simulink library "afa"  (Simulink 8.1)
settings: Solver=ode45  StartTime=0.0  StopTime=10.0  RelTol=1e-3
undefined symbols (not defined in the file or in its folder): ENUM_FCWSTATE_DBS, FALSE, KFCW_DefaultDBSDecel_mps2, KFCW_HapticOnDecelVal_mps2, KFCW_HoldModeLimitSpeed_kph, KFCW_MaxDBSDeceleration_mps2, KFCW_MinDBSDeceleration_mps2, KFCW_WarnLightsDecel_mps2, KFCW_WarnLightSpeedThresh_kph, ZERO_FLOAT
libraries: hcu_lib x2
settings Model: Creator=xsellart  LastModifiedBy=tescamilla

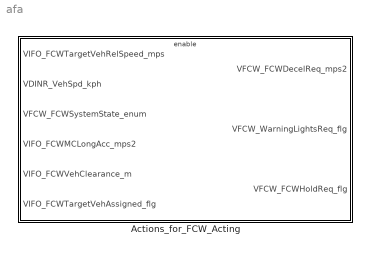
== system afa ==
  Actions_for_FCW_Acting : Subsystem  TreatAsAtomicUnit=on

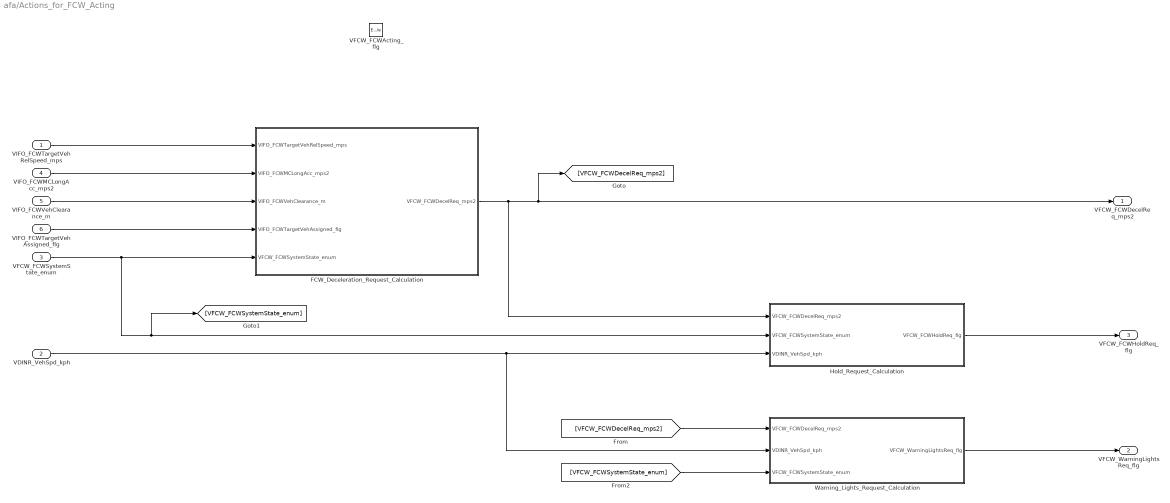
== system afa/Actions_for_FCW_Acting ==
  VIFO_FCWTargetVehRelSpeed_mps : Inport
  VDINR_VehSpd_kph : Inport  Port=2
  VFCW_FCWSystemState_enum : Inport  Port=3
  VIFO_FCWMCLongAcc_mps2 : Inport  Port=4
  VIFO_FCWVehClearance_m : Inport  Port=5
  VIFO_FCWTargetVehAssigned_flg : Inport  Port=6
  VFCW_FCWActing_flg : EnablePort  StatesWhenEnabling=reset
      settings: AttributesFormatString=State=%<StatesWhenEnabling>
  FCW_Deceleration_Request_Calculation : Subsystem
  Hold_Request_Calculation : Subsystem
  Warning_Lights_Request_Calculation : Subsystem
  VFCW_FCWDecelReq_mps2 : Outport  OutputWhenDisabled=reset  InitialOutput=ZERO_FLOAT
  VFCW_WarningLightsReq_flg : Outport  Port=2  OutputWhenDisabled=reset  InitialOutput=FALSE
  VFCW_FCWHoldReq_flg : Outport  Port=3  OutputWhenDisabled=reset  InitialOutput=FALSE
  wires:
  Warning_Lights_Request_Calculation/1(VFCW_WarningLightsReq_flg) -> VFCW_WarningLightsReq_flg/1
  VDINR_VehSpd_kph/1 -> Warning_Lights_Request_Calculation/2(VDINR_VehSpd_kph), Hold_Request_Calculation/3(VDINR_VehSpd_kph)
  VIFO_FCWTargetVehRelSpeed_mps/1 -> FCW_Deceleration_Request_Calculation/1(VIFO_FCWTargetVehRelSpeed_mps)
  Hold_Request_Calculation/1(VFCW_FCWHoldReq_flg) -> VFCW_FCWHoldReq_flg/1
  FCW_Deceleration_Request_Calculation/1(VFCW_FCWDecelReq_mps2) -> VFCW_FCWDecelReq_mps2/1, [VFCW_FCWDecelReq_mps2], Hold_Request_Calculation/1(VFCW_FCWDecelReq_mps2)
  VFCW_FCWSystemState_enum/1 -> [VFCW_FCWSystemState_enum], Hold_Request_Calculation/2(VFCW_FCWSystemState_enum), FCW_Deceleration_Request_Calculation/5(VFCW_FCWSystemState_enum)
  [VFCW_FCWDecelReq_mps2] -> Warning_Lights_Request_Calculation/1(VFCW_FCWDecelReq_mps2)
  [VFCW_FCWSystemState_enum] -> Warning_Lights_Request_Calculation/3(VFCW_FCWSystemState_enum)
  VIFO_FCWMCLongAcc_mps2/1 -> FCW_Deceleration_Request_Calculation/2(VIFO_FCWMCLongAcc_mps2)
  VIFO_FCWVehClearance_m/1 -> FCW_Deceleration_Request_Calculation/3(VIFO_FCWVehClearance_m)
  VIFO_FCWTargetVehAssigned_flg/1 -> FCW_Deceleration_Request_Calculation/4(VIFO_FCWTargetVehAssigned_flg)

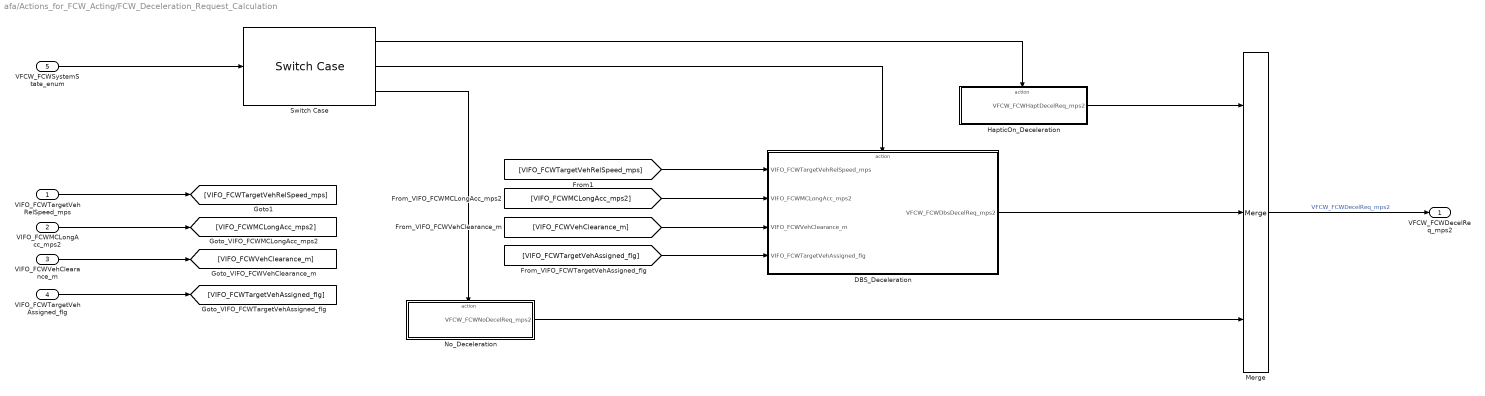
== system afa/Actions_for_FCW_Acting/FCW_Deceleration_Request_Calculation ==
  VIFO_FCWTargetVehRelSpeed_mps : Inport
  VIFO_FCWMCLongAcc_mps2 : Inport  Port=2
  VIFO_FCWVehClearance_m : Inport  Port=3
  VIFO_FCWTargetVehAssigned_flg : Inport  Port=4
  VFCW_FCWSystemState_enum : Inport  Port=5
  DBS_Deceleration : Subsystem  TreatAsAtomicUnit=on
  HapticOn_Deceleration : Subsystem  TreatAsAtomicUnit=on
  Merge : Merge  Inputs=3
  No_Deceleration : Subsystem  TreatAsAtomicUnit=on
  Switch Case : SwitchCase  CaseConditions={5, 7}
  VFCW_FCWDecelReq_mps2 : Outport  OutDataTypeStr=single
  wires:
  VFCW_FCWSystemState_enum/1 -> Switch Case/1
  Switch Case/1 -> HapticOn_Deceleration/Action
  Switch Case/2 -> DBS_Deceleration/Action
  VIFO_FCWTargetVehRelSpeed_mps/1 -> [VIFO_FCWTargetVehRelSpeed_mps]
  [VIFO_FCWTargetVehRelSpeed_mps] -> DBS_Deceleration/1(VIFO_FCWTargetVehRelSpeed_mps)
  Switch Case/3 -> No_Deceleration/Action
  HapticOn_Deceleration/1(VFCW_FCWHaptDecelReq_mps2) -> Merge/1
  DBS_Deceleration/1(VFCW_FCWDbsDecelReq_mps2) -> Merge/2
  No_Deceleration/1(VFCW_FCWNoDecelReq_mps2) -> Merge/3
  Merge/1 -> VFCW_FCWDecelReq_mps2/1  "VFCW_FCWDecelReq_mps2"
  [VIFO_FCWMCLongAcc_mps2] -> DBS_Deceleration/2(VIFO_FCWMCLongAcc_mps2)
  VIFO_FCWMCLongAcc_mps2/1 -> [VIFO_FCWMCLongAcc_mps2]
  VIFO_FCWVehClearance_m/1 -> [VIFO_FCWVehClearance_m]
  [VIFO_FCWVehClearance_m] -> DBS_Deceleration/3(VIFO_FCWVehClearance_m)
  [VIFO_FCWTargetVehAssigned_flg] -> DBS_Deceleration/4(VIFO_FCWTargetVehAssigned_flg)
  VIFO_FCWTargetVehAssigned_flg/1 -> [VIFO_FCWTargetVehAssigned_flg]

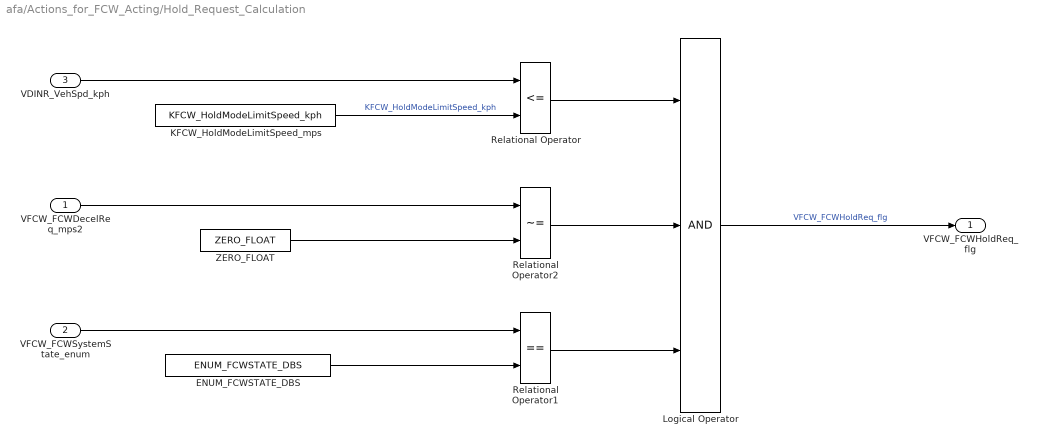
== system afa/Actions_for_FCW_Acting/Hold_Request_Calculation ==
  VFCW_FCWDecelReq_mps2 : Inport
  VFCW_FCWSystemState_enum : Inport  Port=2
  VDINR_VehSpd_kph : Inport  Port=3
  ENUM_FCWSTATE_DBS : Constant  Value=ENUM_FCWSTATE_DBS  OutDataTypeStr=uint8
  KFCW_HoldModeLimitSpeed_mps : Constant  Value=KFCW_HoldModeLimitSpeed_kph  OutDataTypeStr=single
  Logical Operator : Logic  Inputs=3  AllPortsSameDT=off  OutDataTypeStr=boolean
  Relational Operator : RelationalOperator  Operator=<=  OutDataTypeStr=boolean
  Relational Operator1 : RelationalOperator  Operator===  OutDataTypeStr=boolean
  Relational Operator2 : RelationalOperator  Operator=~=  OutDataTypeStr=boolean
  ZERO_FLOAT : Constant  Value=ZERO_FLOAT  OutDataTypeStr=single
  VFCW_FCWHoldReq_flg : Outport
  wires:
  KFCW_HoldModeLimitSpeed_mps/1 -> Relational Operator/2  "KFCW_HoldModeLimitSpeed_kph"
  VDINR_VehSpd_kph/1 -> Relational Operator/1
  ENUM_FCWSTATE_DBS/1 -> Relational Operator1/2
  VFCW_FCWSystemState_enum/1 -> Relational Operator1/1
  Relational Operator2/1 -> Logical Operator/2
  Relational Operator1/1 -> Logical Operator/3
  Logical Operator/1 -> VFCW_FCWHoldReq_flg/1  "VFCW_FCWHoldReq_flg"
  ZERO_FLOAT/1 -> Relational Operator2/2
  VFCW_FCWDecelReq_mps2/1 -> Relational Operator2/1
  Relational Operator/1 -> Logical Operator/1

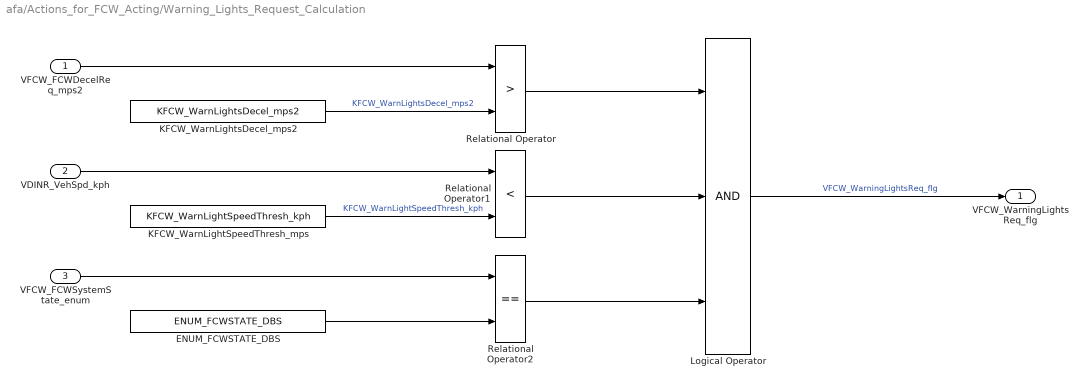
== system afa/Actions_for_FCW_Acting/Warning_Lights_Request_Calculation ==
  VFCW_FCWDecelReq_mps2 : Inport
  VDINR_VehSpd_kph : Inport  Port=2
  VFCW_FCWSystemState_enum : Inport  Port=3
  ENUM_FCWSTATE_DBS : Constant  Value=ENUM_FCWSTATE_DBS  OutDataTypeStr=uint8
  KFCW_WarnLightSpeedThresh_mps : Constant  Value=KFCW_WarnLightSpeedThresh_kph
  KFCW_WarnLightsDecel_mps2 : Constant  Value=KFCW_WarnLightsDecel_mps2
  Logical Operator : Logic  Inputs=3  AllPortsSameDT=off  OutDataTypeStr=boolean
  Relational Operator : RelationalOperator  Operator=>  OutDataTypeStr=boolean
  Relational Operator1 : RelationalOperator  Operator=<  OutDataTypeStr=boolean
  Relational Operator2 : RelationalOperator  Operator===  OutDataTypeStr=boolean
  VFCW_WarningLightsReq_flg : Outport  OutputWhenDisabled=reset  InitialOutput=FALSE
  wires:
  KFCW_WarnLightsDecel_mps2/1 -> Relational Operator/2  "KFCW_WarnLightsDecel_mps2"
  VFCW_FCWDecelReq_mps2/1 -> Relational Operator/1
  KFCW_WarnLightSpeedThresh_mps/1 -> Relational Operator1/2  "KFCW_WarnLightSpeedThresh_kph"
  VDINR_VehSpd_kph/1 -> Relational Operator1/1
  Relational Operator/1 -> Logical Operator/1
  Relational Operator1/1 -> Logical Operator/2
  Logical Operator/1 -> VFCW_WarningLightsReq_flg/1  "VFCW_WarningLightsReq_flg"
  VFCW_FCWSystemState_enum/1 -> Relational Operator2/1
  ENUM_FCWSTATE_DBS/1 -> Relational Operator2/2
  Relational Operator2/1 -> Logical Operator/3

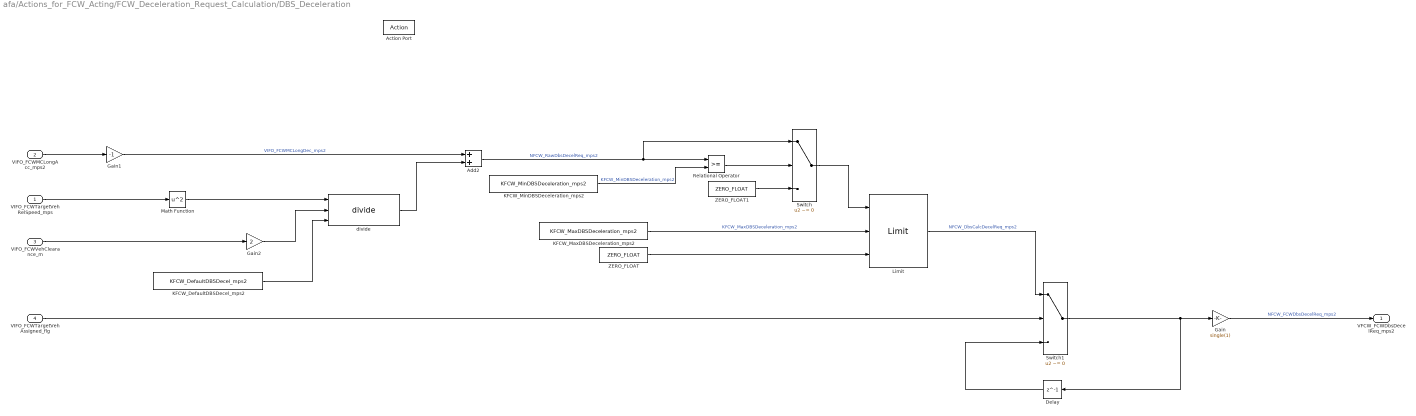
== system afa/Actions_for_FCW_Acting/FCW_Deceleration_Request_Calculation/DBS_Deceleration ==
  VIFO_FCWTargetVehRelSpeed_mps : Inport
  VIFO_FCWMCLongAcc_mps2 : Inport  Port=2
  VIFO_FCWVehClearance_m : Inport  Port=3
  VIFO_FCWTargetVehAssigned_flg : Inport  Port=4
  Action Port : ActionPort  ActionType=case
  Add2 : Sum
  Delay : Delay  DelayLength=1  InitialCondition=0
  Gain : Gain  Gain=single(1)
  Gain1 : Gain  Gain=-1
  Gain2 : Gain  Gain=2
  KFCW_DefaultDBSDecel_mps2 : Constant  Value=KFCW_DefaultDBSDecel_mps2
  KFCW_MaxDBSDeceleration_mps2 : Constant  Value=KFCW_MaxDBSDeceleration_mps2
  KFCW_MinDBSDeceleration_mps2 : Constant  Value=KFCW_MinDBSDeceleration_mps2
  Limit : hcu_lib/Limit  SystemSampleTime=-1
  Math Function : Math  Operator=square  SaturateOnIntegerOverflow=on
  Relational Operator : RelationalOperator  OutDataTypeStr=boolean
  Switch : Switch  Criteria=u2 ~= 0
  Switch1 : Switch  Criteria=u2 ~= 0
  ZERO_FLOAT : Constant  Value=ZERO_FLOAT
  ZERO_FLOAT1 : Constant  Value=ZERO_FLOAT
  divide : hcu_lib/divide
  VFCW_FCWDbsDecelReq_mps2 : Outport
  wires:
  ZERO_FLOAT/1 -> Limit/3
  VIFO_FCWTargetVehRelSpeed_mps/1 -> Math Function/1
  KFCW_MaxDBSDeceleration_mps2/1 -> Limit/2  "KFCW_MaxDBSDeceleration_mps2"
  Limit/1 -> Switch1/1  "NFCW_DbsCalcDecelReq_mps2"
  VIFO_FCWMCLongAcc_mps2/1 -> Gain1/1
  Math Function/1 -> divide/1
  VIFO_FCWVehClearance_m/1 -> Gain2/1
  Gain2/1 -> divide/2
  KFCW_DefaultDBSDecel_mps2/1 -> divide/3
  Gain1/1 -> Add2/1  "VIFO_FCWMCLongDec_mps2"
  divide/1 -> Add2/2
  Add2/1 -> Switch/1, Relational Operator/1  "NFCW_RawDbsDecelReq_mps2"
  KFCW_MinDBSDeceleration_mps2/1 -> Relational Operator/2  "KFCW_MinDBSDeceleration_mps2"
  Relational Operator/1 -> Switch/2
  ZERO_FLOAT1/1 -> Switch/3
  Switch/1 -> Limit/1
  VIFO_FCWTargetVehAssigned_flg/1 -> Switch1/2
  Switch1/1 -> Delay/1, Gain/1
  Delay/1 -> Switch1/3
  Gain/1 -> VFCW_FCWDbsDecelReq_mps2/1  "NFCW_FCWDbsDecelReq_mps2"

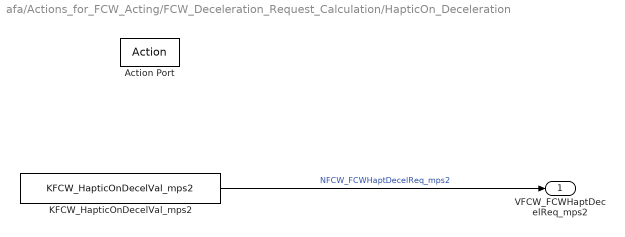
== system afa/Actions_for_FCW_Acting/FCW_Deceleration_Request_Calculation/HapticOn_Deceleration ==
  Action Port : ActionPort  ActionType=case
  KFCW_HapticOnDecelVal_mps2 : Constant  Value=KFCW_HapticOnDecelVal_mps2  OutDataTypeStr=single
  VFCW_FCWHaptDecelReq_mps2 : Outport
  wires:
  KFCW_HapticOnDecelVal_mps2/1 -> VFCW_FCWHaptDecelReq_mps2/1  "NFCW_FCWHaptDecelReq_mps2"

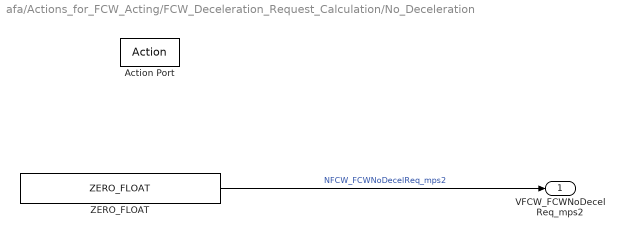
== system afa/Actions_for_FCW_Acting/FCW_Deceleration_Request_Calculation/No_Deceleration ==
  Action Port : ActionPort  ActionType=default
  ZERO_FLOAT : Constant  Value=ZERO_FLOAT  OutDataTypeStr=single
  VFCW_FCWNoDecelReq_mps2 : Outport
  wires:
  ZERO_FLOAT/1 -> VFCW_FCWNoDecelReq_mps2/1  "NFCW_FCWNoDecelReq_mps2"
